simulink model "stackercrane_singlemass_experimentdesign"  (R2017a)
settings: Solver=ode45  StartTime=0.0  StopTime=30  MaxStep=0.02  RelTol=1e-3  EnableMultiTasking=on
libraries: simulink x1
settings Model: Creator=beck  LastModifiedBy=xk2337
settings DataIOCC: LimitDataPoints=on  SaveFormat=Array  SignalLoggingSaveFormat=ModelDataLogs
settings OptimizationCC: ExpressionDepthLimit=2147483647  InitFltsAndDblsToZero=on  LifeSpan=inf
settings DebuggingCC: SaveWithParameterizedLinksMsg=none  UnderspecifiedInitializationDetection=Classic  MergeDetectMultiDrivingBlocksExec=none  SignalResolutionControl=TryResolveAllWithWarning  SolverPrmCheckMsg=warning  FcnCallInpInsideContextMsg=warning  StateNameClashWarn=warning  SFUnexpectedBacktrackingDiag=warning  SFNoUnconditionalDefaultTransitionDiag=warning  SFExecutionAtInitializationDiag=none
settings HardwareCC: ProdBitPerPointer=32  ProdBitPerSizeT=32  ProdBitPerPtrDiffT=32  ProdLargestAtomicFloat=None  ProdIntDivRoundTo=Undefined  ProdEndianess=Unspecified  ProdWordSize=32  ProdHWDeviceType=32-bit Generic
settings ModelReferenceCC: PropagateSignalLabelsOutOfModel=off
settings GRTTargetCC: TargetFcnLib=ansi_tfl_tmw.mat  TargetLangStandard=C89/C90 (ANSI)  GeneratePreprocessorConditionals=Disable all  CombineOutputUpdateFcns=off  GRTInterface=on
settings ConfigComp: CovMetricSettings=dw  CovHtmlReporting=on  CovSaveCumulativeToWorkspaceVar=on  CovSaveSingleToWorkspaceVar=on  CovExternalEMLEnable=off

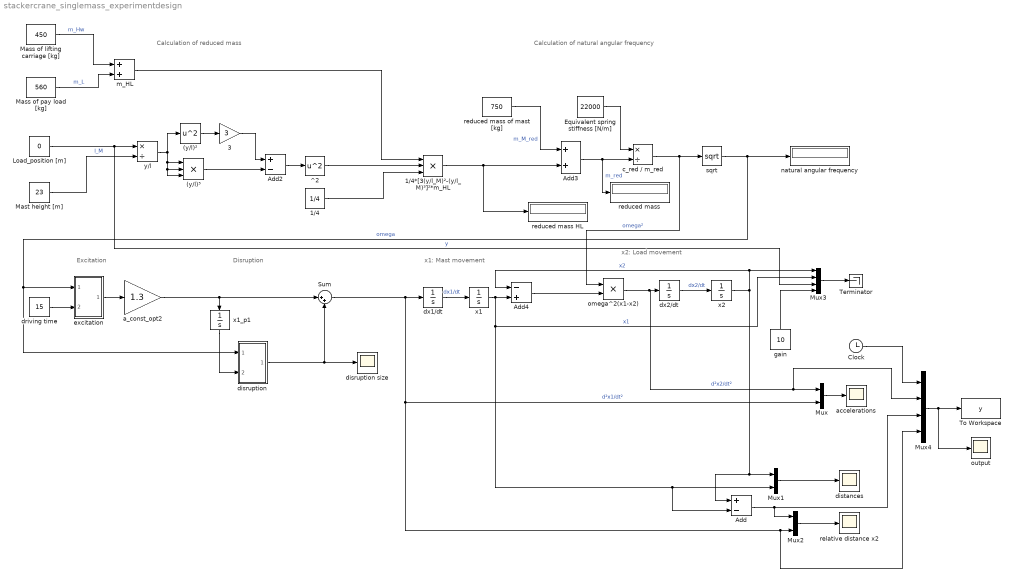
== system stackercrane_singlemass_experimentdesign ==
  note: Calculation of natural angular frequency
  note: Calculation of reduced mass
  note: x1: Mast movement
  note: x2: Load movement
  note: Excitation
  note: Disruption
  (y/l)² : Math  Operator=square  SaturateOnIntegerOverflow=on
  (y/l)³ : Product  Inputs=3  RndMeth=Zero
  1/4 : Constant  Value=1/4
  1/4*[3(y/l_M)²-(y/l_M)³]²*m_HL : Product  Inputs=3  RndMeth=Zero
  3 : Gain  Gain=3
  Add : Sum  Inputs=+-
  Add2 : Sum  Inputs=+-
  Add3 : Sum
  Add4 : Sum  Inputs=-+
  Clock : Clock
  Equivalent spring stiffness [N/m] : Constant  Value=22000
  Load_position [m] : Constant  Value=0
  Mass of lifting carriage [kg] : Constant  Value=450
  Mass of pay load [kg] : Constant  Value=560
  Mast height [m] : Constant  Value=23
  Mux : Mux  Inputs=2
  Mux1 : Mux  Inputs=2
  Mux2 : Mux  Inputs=2
  Mux3 : Mux
  Mux4 : Mux
  Sum : Sum  Inputs=|++
  Terminator : Terminator
  To Workspace : ToWorkspace  VariableName=y  SampleTime=-1
  ^2 : Math  Operator=square  SaturateOnIntegerOverflow=on
  a_const_opt2 : Gain  Gain=1.3
  accelerations : Scope
  c_red / m_red : Product  Inputs=*/  RndMeth=Zero
  disruption : Subsystem
  disruption size : Scope
  distances : Scope
  driving time : Constant  Value=15
  dx1/dt : Integrator
  dx2/dt : Integrator
  excitation : Subsystem
  gain : Constant  Value=10
  m_HL : Sum
  natural angular frequency : Display
  omega^2(x1-x2) : Product  RndMeth=Zero
  output : Scope
  reduced mass : Display
  reduced mass HL : Display
  reduced mass of mast [kg] : Constant  Value=750
  relative distance x2 : Scope
  sqrt : Math  Operator=sqrt  SaturateOnIntegerOverflow=on
  x1 : Integrator
  x1_p1 : Integrator
  x2 : Integrator
  y/l : Product  Inputs=*/  RndMeth=Zero
  wires:
  Load_position [m]/1 -> y/l/1, Mux3/3  "y"
  Mux/1 -> accelerations/1
  Mux1/1 -> distances/1
  Mast height [m]/1 -> y/l/2  "l_M"
  (y/l)²/1 -> 3/1
  3/1 -> Add2/1
  (y/l)³/1 -> Add2/2
  y/l/1 -> (y/l)³/1, (y/l)³/2, (y/l)³/3, (y/l)²/1
  Equivalent spring stiffness [N/m]/1 -> c_red / m_red/1
  c_red / m_red/1 -> sqrt/1, omega^2(x1-x2)/1  "omega²"
  Add3/1 -> reduced mass/1, c_red / m_red/2  "m_red"
  sqrt/1 -> natural angular frequency/1, disruption/1(In1), excitation/1(In1)  "omega"
  omega^2(x1-x2)/1 -> dx2/dt/1, Mux/1, Mux4/2  "d²x2/dt²"
  dx2/dt/1 -> x2/1  "dx2/dt"
  dx1/dt/1 -> x1/1  "dx1/dt"
  Add4/1 -> omega^2(x1-x2)/2
  x1/1 -> Add4/2, Mux3/2, Mux1/2, Add/2  "x1"
  x2/1 -> Add4/1, Mux3/1, Add/1, Mux1/1  "x2"
  gain/1 -> Mux3/4
  Add2/1 -> ^2/1
  reduced mass of mast [kg]/1 -> Add3/1  "m_M_red"
  Mux2/1 -> relative distance x2/1
  Add/1 -> Mux4/3, Mux2/1
  Mass of pay load [kg]/1 -> m_HL/2  "m_L"
  Mass of lifting carriage [kg]/1 -> m_HL/1  "m_Hw"
  1/4*[3(y/l_M)²-(y/l_M)³]²*m_HL/1 -> Add3/2, reduced mass HL/1
  ^2/1 -> 1/4*[3(y/l_M)²-(y/l_M)³]²*m_HL/2
  m_HL/1 -> 1/4*[3(y/l_M)²-(y/l_M)³]²*m_HL/1
  1/4/1 -> 1/4*[3(y/l_M)²-(y/l_M)³]²*m_HL/3
  Sum/1 -> dx1/dt/1, Mux/2, Mux2/2, Mux4/4  "d²x1/dt²"
  excitation/1(Out1) -> a_const_opt2/1
  disruption/1(Out1) -> disruption size/1, Sum/2
  Clock/1 -> Mux4/1
  Mux4/1 -> To Workspace/1, output/1
  a_const_opt2/1 -> Sum/1, x1_p1/1
  x1_p1/1 -> disruption/2(In2)
  Mux3/1 -> Terminator/1
  driving time/1 -> excitation/2(In2)

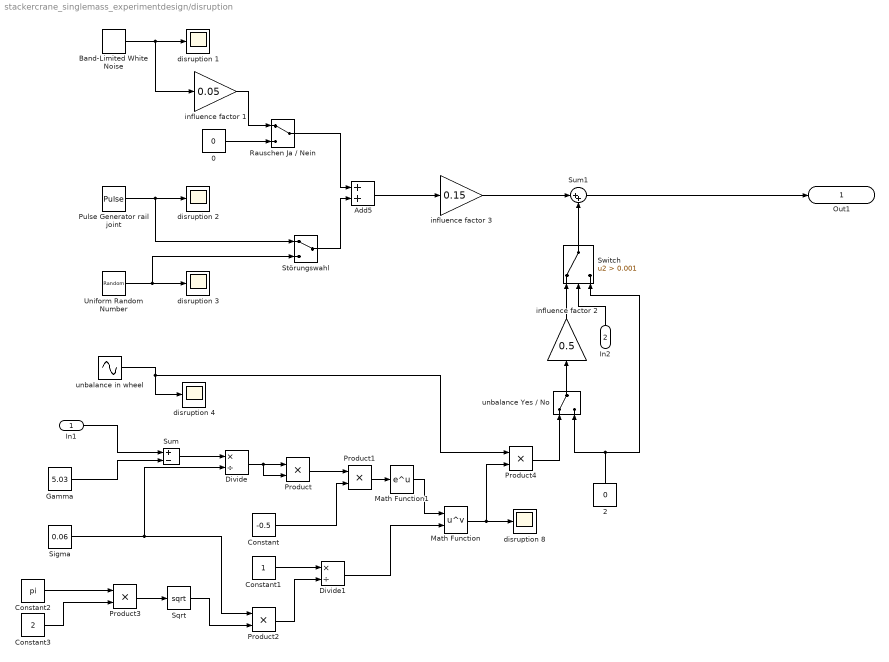
== system stackercrane_singlemass_experimentdesign/disruption ==
  In1 : Inport
  In2 : Inport  Port=2
  0 : Constant  Value=0
  2 : Constant  Value=0
  Add5 : Sum
  Band-Limited White Noise : simulink/Sources/Band-Limited White Noise  Cov=[0.1]  Ts=0.1  seed=[23341]
  Constant : Constant  Value=-0.5
  Constant1 : Constant
  Constant2 : Constant  Value=pi
  Constant3 : Constant  Value=2
  Divide : Product  Inputs=*/
  Divide1 : Product  Inputs=*/
  Gamma : Constant  Value=5.03
  Math Function : Math  Operator=pow  SaturateOnIntegerOverflow=on
  Math Function1 : Math  SaturateOnIntegerOverflow=on
  Product{,1..4} (5 alike) : Product  RndMeth=Zero
  Pulse Generator rail joint : DiscretePulseGenerator  PulseType=Time based  Amplitude=-1  Period=4
  Rauschen Ja / Nein : ManualSwitch
  Sigma : Constant  Value=0.06
  Sqrt : Sqrt  SaturateOnIntegerOverflow=on
  Störungswahl : ManualSwitch
  Sum : Sum  Inputs=+-
  Sum1 : Sum  Inputs=|++
  Switch : Switch  Criteria=u2 > Threshold  Threshold=0.001
  Uniform Random Number : UniformRandomNumber  SampleTime=1
  disruption {1..4,8} (5 alike) : Scope
  influence factor 1 : Gain  Gain=0.05
  influence factor 2 : Gain  Gain=0.5
  influence factor 3 : Gain  Gain=0.15
  unbalance Yes / No : ManualSwitch
  unbalance in wheel : Sin  Frequency=5  SampleTime=0
  Out1 : Outport
  wires:
  Pulse Generator rail joint/1 -> disruption 2/1, Störungswahl/1
  Add5/1 -> influence factor 3/1
  Band-Limited White Noise/1 -> disruption 1/1, influence factor 1/1
  Störungswahl/1 -> Add5/2
  Uniform Random Number/1 -> disruption 3/1, Störungswahl/2
  Rauschen Ja / Nein/1 -> Add5/1
  unbalance in wheel/1 -> disruption 4/1, Product4/1
  Gamma/1 -> Sum/2
  Sum/1 -> Divide/1
  Sigma/1 -> Divide/2, Product2/1
  Divide/1 -> Product/1, Product/2
  Product/1 -> Product1/1
  Constant/1 -> Product1/2
  Constant1/1 -> Divide1/1
  Constant2/1 -> Product3/1
  Constant3/1 -> Product3/2
  Product3/1 -> Sqrt/1
  Sqrt/1 -> Product2/2
  Product2/1 -> Divide1/2
  Math Function/1 -> Product4/2, disruption 8/1
  Product1/1 -> Math Function1/1
  Math Function1/1 -> Math Function/1
  Divide1/1 -> Math Function/2
  2/1 -> Switch/3, unbalance Yes / No/2
  Product4/1 -> unbalance Yes / No/1
  In1/1 -> Sum/1
  influence factor 3/1 -> Sum1/1
  unbalance Yes / No/1 -> influence factor 2/1
  Sum1/1 -> Out1/1
  influence factor 2/1 -> Switch/1
  In2/1 -> Switch/2
  Switch/1 -> Sum1/2
  influence factor 1/1 -> Rauschen Ja / Nein/1
  0/1 -> Rauschen Ja / Nein/2

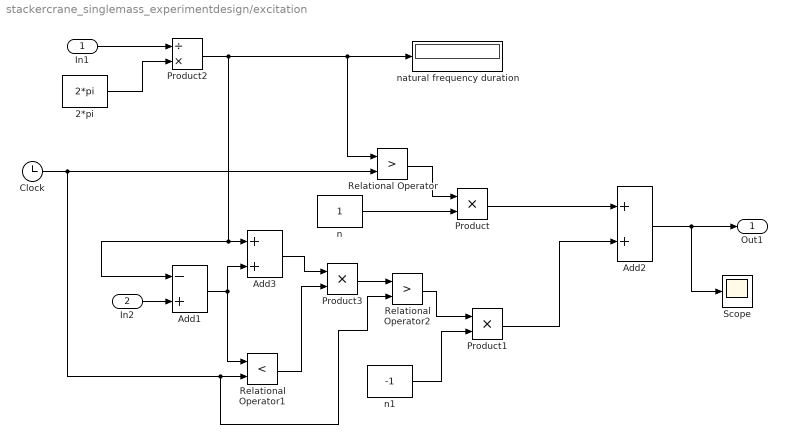
== system stackercrane_singlemass_experimentdesign/excitation ==
  In1 : Inport
  In2 : Inport  Port=2
  2*pi : Constant  Value=2*pi
  Add1 : Sum  Inputs=-+
  Add2 : Sum
  Add3 : Sum
  Clock : Clock
  Product : Product  RndMeth=Zero
  Product1 : Product  RndMeth=Zero
  Product2 : Product  Inputs=/*  RndMeth=Zero
  Product3 : Product  RndMeth=Zero
  Relational Operator : RelationalOperator  Operator=>  RndMeth=Nearest
  Relational Operator1 : RelationalOperator  Operator=<  RndMeth=Nearest
  Relational Operator2 : RelationalOperator  Operator=>  RndMeth=Nearest
  Scope : Scope
  n : Constant
  n1 : Constant  Value=-1
  natural frequency duration : Display
  Out1 : Outport
  wires:
  2*pi/1 -> Product2/2
  Clock/1 -> Relational Operator/2, Relational Operator2/2, Relational Operator1/2
  n/1 -> Product/2
  Product2/1 -> natural frequency duration/1, Relational Operator/1, Add1/1, Add3/1
  Relational Operator/1 -> Product/1
  In1/1 -> Product2/1
  Add2/1 -> Out1/1, Scope/1
  Product/1 -> Add2/1
  n1/1 -> Product1/2
  Relational Operator2/1 -> Product1/1
  Add3/1 -> Product3/1
  Relational Operator1/1 -> Product3/2
  Product3/1 -> Relational Operator2/1
  Product1/1 -> Add2/2
  In2/1 -> Add1/2
  Add1/1 -> Relational Operator1/1, Add3/2
